simulink model "model_T_PSH_IEEE39"  (R2020b)
settings: Solver=ode3  StartTime=0.0  StopTime=300  FixedStep=Ts  RelTol=1e-3
PostLoadFcn:
  | IEEE39BusLineLength;
  | vNomHV = 345E3;fNom=60;load('Dynamicload.mat');
InitFcn:
  | IEEE39BusLineLength;
  | vNomHV = 345E3;fNom=60;load('Dynamicload.mat');
values from neighbouring files (symbols this model uses):
  At = 1.48    [MAIN_T_PSH_IEEE39.m]
  Dturb = 0.3    [MAIN_T_PSH_IEEE39.m]
  fix_mode = 1    [MAIN_T_PSH_IEEE39.m]
  Gmax = 1    [MAIN_T_PSH_IEEE39.m]
  Gmin = 0    [MAIN_T_PSH_IEEE39.m]
  Hdam = 1    [MAIN_T_PSH_IEEE39.m]
  Kd = 1    [MAIN_T_PSH_IEEE39.m]    (also in plots_T_PSH_IEEE39.m)
  max_delay_gen2pump = 20    [MAIN_T_PSH_IEEE39.m]
  max_delay_pump2hsc = 30    [MAIN_T_PSH_IEEE39.m]
  pgen_pump = Kd*Pref    (= 0.9)    [MAIN_T_PSH_IEEE39.m]
  pgen_turb = (1-Kd)*Pref    (= 0)    [MAIN_T_PSH_IEEE39.m]
  pgen_turb_gen2pump = (1-kd_gen2pump)*Pref    (= 0)    [MAIN_T_PSH_IEEE39.m]
  pgen_turb_hsc2gen = (1-kd_hsc2gen)*Pref    (= 0.36)    [MAIN_T_PSH_IEEE39.m]
  pgen_turb_pump2hsc = (1-kd_pump2hsc)*Pref    (= 0.36)    [MAIN_T_PSH_IEEE39.m]
  Pref = 0.9    [MAIN_T_PSH_IEEE39.m]    (also in MAIN_VS_PSH.m = 1)
  qNL = 0.1    [MAIN_T_PSH_IEEE39.m]
  R = 0.04    [MAIN_T_PSH_IEEE39.m]
  r = 0.31    [MAIN_T_PSH_IEEE39.m]
  Rp = 0.05    [IEEE39BusLineLength.m]
  Sn = 320E6    (= 320000000)    [MAIN_T_PSH_IEEE39.m]
  t_gen2pump = 10    [MAIN_T_PSH_IEEE39.m]
  t_hsc2gen = 150    [MAIN_T_PSH_IEEE39.m]
  t_pump2hsc = 35    [MAIN_T_PSH_IEEE39.m]
  t_sw_off = 220    [MAIN_FS_PSH_IEEE39.m]    (also in MAIN_T_PSH_IEEE39.m; MAIN_VS_PSH.m = 45)
  t_sw_on = 130    [MAIN_FS_PSH_IEEE39.m]    (also in MAIN_T_PSH_IEEE39.m; MAIN_VS_PSH.m = 35)
  Tf = 0.05    [MAIN_T_PSH_IEEE39.m]
  Tg = 0.5    [MAIN_T_PSH_IEEE39.m]
  TL_10_11_len = 14    [IEEE39BusLineLength.m]
  TL_10_13_len = 14    [IEEE39BusLineLength.m]
  TL_13_14_len = 32    [IEEE39BusLineLength.m]
  TL_14_15_len = 70    [IEEE39BusLineLength.m]
  TL_15_16_len = 31.5    [IEEE39BusLineLength.m]
  TL_16_17_len = 26    [IEEE39BusLineLength.m]
  TL_16_19_len = 61    [IEEE39BusLineLength.m]
  TL_16_21_len = 46    [IEEE39BusLineLength.m]
  TL_16_24_len = 15    [IEEE39BusLineLength.m]
  TL_17_18_len = 26    [IEEE39BusLineLength.m]
  TL_17_27_len = 59    [IEEE39BusLineLength.m]
  TL_1_2_len = 134    [IEEE39BusLineLength.m]
  TL_1_39_len = 105    [IEEE39BusLineLength.m]
  TL_21_22_len = 47    [IEEE39BusLineLength.m]
  TL_22_23_len = 33    [IEEE39BusLineLength.m]
  TL_24_23_len = 88    [IEEE39BusLineLength.m]
  TL_25_26_len = 101    [IEEE39BusLineLength.m]
  TL_26_27_len = 46.5    [IEEE39BusLineLength.m]
  TL_26_28_len = 151    [IEEE39BusLineLength.m]
  TL_26_29_len = 200    [IEEE39BusLineLength.m]
  TL_28_29_len = 48    [IEEE39BusLineLength.m]
  TL_2_25_len = 28    [IEEE39BusLineLength.m]
  TL_2_2_len = 49    [IEEE39BusLineLength.m]
  TL_3_18_len = 42    [IEEE39BusLineLength.m]
  TL_3_4_len = 53    [IEEE39BusLineLength.m]
  TL_4_14_len = 33    [IEEE39BusLineLength.m]
  TL_4_5_len = 32.5    [IEEE39BusLineLength.m]
  TL_5_6_len = 14    [IEEE39BusLineLength.m]
  TL_5_8_len = 32    [IEEE39BusLineLength.m]
  TL_6_11_len = 26.5    [IEEE39BusLineLength.m]
  TL_6_7_len = 25.5    [IEEE39BusLineLength.m]
  TL_7_8_len = 15    [IEEE39BusLineLength.m]
  TL_8_9_len = 93    [IEEE39BusLineLength.m]
  TL_9_39_len = 136    [IEEE39BusLineLength.m]
  Tr = 6.88    [MAIN_T_PSH_IEEE39.m]
  Ts = 25e-6    (= 2.5e-05)    [MAIN_FS_PSH_IEEE39.m]    (also in MAIN_T_PSH_IEEE39.m; MAIN_VS_PSH.m = 1e-07)
  Velm = 0.05    [MAIN_T_PSH_IEEE39.m]
  Vn = 18000    [MAIN_T_PSH_IEEE39.m]
undefined symbols (not defined in the file or in its folder): D1, Delta, load15, load16, load18, load20, load21, load23, load24, load25, load26, load27, load28, load29, load3, load39, load4, load7, load8
libraries: powerlib x216, sps_avr x10, simulink_extras x7, powerlib_meascontrol x5, simulink x1
(part 5 of 9)

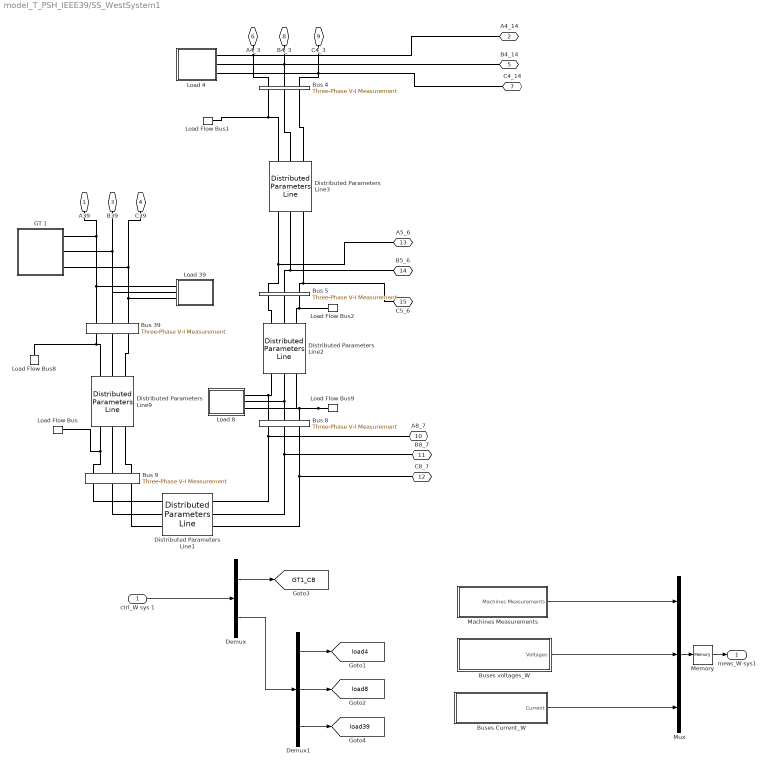
== system model_T_PSH_IEEE39/SS_WestSystem1 ==
  ctrl_W sys 1 : Inport
  Bus 39 : powerlib/Measurements/Three-Phase V-I Measurement  VoltageMeasurement=phase-to-ground  SetLabelV=on  LabelV=V_bus_39  Vpu=off  VpuLL=off  CurrentMeasurement=yes  SetLabelI=on  LabelI=I_bus_39  Ipu=off  Pbase=100e6  Vbase=345e3  OutputType=Complex  PhasorSimulation=off  PSBequivalent=0
  Bus 4 : powerlib/Measurements/Three-Phase V-I Measurement  VoltageMeasurement=phase-to-ground  SetLabelV=on  LabelV=V_bus_4  Vpu=off  VpuLL=off  CurrentMeasurement=yes  SetLabelI=on  LabelI=I_bus_4  Ipu=off  Pbase=100e6  Vbase=230e3  OutputType=Complex  PhasorSimulation=off  PSBequivalent=0
  Bus 5 : powerlib/Measurements/Three-Phase V-I Measurement  VoltageMeasurement=phase-to-ground  SetLabelV=on  LabelV=V_bus_5  Vpu=off  VpuLL=off  CurrentMeasurement=yes  SetLabelI=on  LabelI=I_bus_5  Ipu=off  Pbase=100e6  Vbase=230e3  OutputType=Complex  PhasorSimulation=off  PSBequivalent=0
  Bus 8 : powerlib/Measurements/Three-Phase V-I Measurement  VoltageMeasurement=phase-to-ground  SetLabelV=on  LabelV=V_bus_8  Vpu=off  VpuLL=off  CurrentMeasurement=yes  SetLabelI=on  LabelI=I_bus_8  Ipu=off  Pbase=100e6  Vbase=230e3  OutputType=Complex  PhasorSimulation=off  PSBequivalent=0
  Bus 9 : powerlib/Measurements/Three-Phase V-I Measurement  VoltageMeasurement=phase-to-ground  SetLabelV=on  LabelV=V_bus_9  Vpu=off  VpuLL=off  CurrentMeasurement=yes  SetLabelI=on  LabelI=I_bus_9  Ipu=off  Pbase=100e6  Vbase=230e3  OutputType=Complex  PhasorSimulation=off  PSBequivalent=0
  Buses Current_W : Subsystem
  Buses voltages_W : Subsystem
  Demux : Demux  Outputs=[1 6]
  Demux1 : Demux  Outputs=[2 2 2]
  Distributed Parameters Line1 : powerlib/Elements/Distributed Parameters Line  Phases=3  Length=TL_8_9_len  Frequency=fNom  Resistance=[2.738 10.95]/TL_8_9_len  Inductance=[0.115 0.344]/TL_8_9_len  Capacitance=[0.848e-6 0.385e-6]/TL_8_9_len  x1=[-0.000375 7.83180070356268e-09 238945.685626359 24258.781932988;-0.00035 7.68853749159509e-09 239163.697394933 22005.7375529596;-0.000325 7.5445913392716e-09 239360.465261036 19750.7384960824;-0.0003 7.39997503272177e-09 239535.971746608 17493.9850644112;-0.000275 7.25470141760213e-09 239690.201262149 15235.6777158346;-0.00025 7.10878339795517e-09 239823.140108101 12976.017046269;-0.000225 6.96223393506311e-09 239934.776476067 10715.2037718408;-0.0002 6.8150660462966e-09 240025.100449859 8453.43871105719;-0.000175 6.66729280395846e-09 240094.10400638 6190.92276696862;-0.00015 6.51892733412251e-09 240141.781016335 3927.85690932335;-0.000125 6.36998281546766e-09 240168.127244777 1664.44215671614;-0.0001 6.22047247810726e-09 240173.14035148 -599.120441267409;-7.5e-05 6.07040960241395e-09 240156.819891152 -2862.62982190919;-5e-05 5.91980751784004e-09 240119.16731347 -5125.88492721818;-2.5e-05 5.76867960173348e-09 240060.185962955 -7388.68472178954]  x2=[-0.000375 6.41970903757356e-09 248393.348574129 9449.4998144962;-0.00035 6.32122932359373e-09 248471.368448558 7108.07301672364;-0.000325 6.2221881214754e-09 248527.317659354 4766.01483880616;-0.0003 6.1225942286308e-09 248561.191236786 2423.53331589312;-0.000275 6.02245649156536e-09 248572.986172007 80.8365207378492;-0.00025 5.92178380509189e-09 248562.701417321 -2261.8674547846;-0.000225 5.82058511154051e-09 248530.337886282 -4604.37051816137;-0.0002 5.71886939996431e-09 248475.898453604 -6946.46459472579;-0.000175 5.61664570534093e-09 248399.387954912 -9287.94164613975;-0.00015 5.51392310776999e-09 248300.813186313 -11628.5936888729;-0.000125 5.41071073166657e-09 248180.182903786 -13968.2128126769;-0.0001 5.30701774495068e-09 248037.50782241 -16306.5911990532;-7.5e-05 5.20285335823298e-09 247872.800615413 -18643.521139713;-5e-05 5.09822682399658e-09 247686.075913039 -20978.7950550263;-2.5e-05 4.99314743577521e-09 247477.350301256 -23312.2055124614]  x3=[-0.000375 -2.80416857734533e-11 994.785547993016 298.958599838395;-0.00035 -2.82588220159761e-11 997.558943228101 289.569860125711;-0.000325 -2.84734481465322e-11 1000.24372950986 280.15539914373;-0.0003 -2.86855451007874e-11 1002.83966836006 270.71605313931;-0.000275 -2.88950940390642e-11 1005.34652919239 261.252660569742;-0.00025 -2.9102076348014e-11 1007.76408933299 251.766062028274;-0.000225 -2.93064736422715e-11 1010.09213404017 242.25710016944;-0.0002 -2.95082677660871e-11 1012.33045652356 232.726619634214;-0.000175 -2.970744079494e-11 1014.47885796241 223.175466974983;-0.00015 -2.990397503713e-11 1016.53714752327 213.604490580353;-0.000125 -3.00978530353495e-11 1018.50514237696 204.014540599786;-0.0001 -3.02890575682336e-11 1020.38266771482 194.406468868091;-7.5e-05 -3.047757165189e-11 1022.16955676417 184.781128829754;-5e-05 -3.0663378541408e-11 1023.8656508032 175.13937546313;-2.5e-05 -3.08464617323452e-11 1025.47079917504 165.482065204505]  x4=[-0.000375 4.48982480771432e-11 315.841922857234 -130.234658424009;-0.00035 4.48725488427444e-11 314.600450218203 -133.205545988237;-0.000325 4.48428637690998e-11 313.331032948132 -136.164601465662;-0.0003 4.48091954930093e-11 312.033783804004 -139.111562015868;-0.000275 4.47715470050838e-11 310.708818014987 -142.046165872778;-0.00025 4.47299216494798e-11 309.356253272204 -144.96815236791;-0.000225 4.46843231236019e-11 307.976209718277 -147.877261953529;-0.0002 4.4634755477775e-11 306.568809936654 -150.7732362257;-0.000175 4.45812231148839e-11 305.13417894072 -153.655817947243;-0.00015 4.45237307899826e-11 303.672444162696 -156.524751070583;-0.000125 4.44622836098719e-11 302.183735442318 -159.379780760491;-0.0001 4.43968870326456e-11 300.6681850153 -162.220653416721;-7.5e-05 4.43275468672058e-11 299.125927501596 -165.04711669654;-5e-05 4.42542692727468e-11 297.557099893435 -167.858919537134;-2.5e-05 4.41770607582085e-11 295.961841543156 -170.655812177918]  x5=0.000363923068793392  V1=ones(3,3)  V2=ones(3,3)  I1=ones(3,3)  I2=ones(3,3)  nHarmo=1  Measurements=None  Decoupling=off  VsMag0=0  VrMag0=0  VsAngle0=0  VrAngle0=0  IsMag0=0  IrMag0=0  IsAngle0=0  IrAngle0=0
  Distributed Parameters Line2 : powerlib/Elements/Distributed Parameters Line  Phases=3  Length=TL_5_8_len  Frequency=fNom  Resistance=[0.952 3.809]/TL_5_8_len  Inductance=[0.035 0.106]/TL_5_8_len  Capacitance=[0.329e-6 0.15e-6]/TL_5_8_len  x1=[-0.00015 6.51892733412251e-09 0 0;-0.000125 6.36998281546766e-09 118642.614431542 -208823.920451668;-0.0001 6.22047247810726e-09 120605.423697804 -207696.480630433;-7.5e-05 6.07040960241395e-09 122557.52009298 -206550.592006867;-5e-05 5.91980751784004e-09 124498.730220582 -205386.356365422;-2.5e-05 5.76867960173348e-09 126428.881651101 -204203.877120241]  x2=[-0.00015 6.93971136599651e-09 0 0;-0.000125 6.78863743170585e-09 127269.929121309 -203855.09967514;-0.0001 6.63696049138591e-09 129185.526033388 -202646.571246844;-7.5e-05 6.48469401785956e-09 131089.647940081 -201420.042578368;-5e-05 6.33185153631539e-09 132982.125706271 -200175.622617078;-2.5e-05 6.17844662310637e-09 134862.791231139 -198913.421899552]  x3=[-0.00015 1.24925992865406e-11 0 0;-0.000125 1.24360709657444e-11 771.064654820684 -1268.89273840881;-0.0001 1.23784380012184e-11 782.98923328193 -1261.56936239942;-7.5e-05 1.23197055122557e-11 794.844262112154 -1254.13392650475;-5e-05 1.22598787158157e-11 806.628688279148 -1246.5870911832;-2.5e-05 1.21989629260604e-11 818.341465022041 -1238.92952678831]  x4=[-0.00015 1.33899500783991e-12 0 0;-0.000125 1.07256616847881e-12 -44.3180796703685 -8.8205638210786;-0.0001 8.06042057588946e-13 -44.2330187586768 -9.23786088668168;-7.5e-05 5.39446349382905e-13 -44.1440288144991 -9.65433739206657;-5e-05 2.7280272443298e-13 -44.0511177424369 -10.0699563433819;-2.5e-05 6.13486756769849e-15 -43.9542937953889 -10.4846808229494]  x5=0.000126095202129185  V1=ones(3,3)  V2=ones(3,3)  I1=ones(3,3)  I2=ones(3,3)  nHarmo=1  Measurements=None  Decoupling=off  VsMag0=0  VrMag0=0  VsAngle0=0  VrAngle0=0  IsMag0=0  IrMag0=0  IsAngle0=0  IrAngle0=0
  Distributed Parameters Line3 : powerlib/Elements/Distributed Parameters Line  Phases=3  Length=TL_4_5_len  Frequency=fNom  Resistance=[0.952 3.809]/TL_4_5_len  Inductance=[0.04 0.121]/TL_4_5_len  Capacitance=[0.299e-6 0.136e-6]/TL_4_5_len  x1=[-0.00015 1.25269920383338e-09 0 0;-0.000125 1.10475045682001e-09 240898.71921355 -2229.53954135192;-0.0001 9.56703579483276e-10 240867.001075201 -4499.8148800452;-7.5e-05 8.08571722202861e-10 240813.887737099 -6769.69051916246;-5e-05 6.60368042906836e-10 240739.383917078 -9038.96483522477;-2.5e-05 5.12105705902926e-10 240643.496232999 -11307.4362581662]  x2=[-0.00015 6.93649042877756e-09 0 0;-0.000125 6.78534623604884e-09 240178.659570335 -8291.44191932873;-0.0001 6.63359932963387e-09 240089.841706274 -10554.6617227481;-7.5e-05 6.48126318857032e-09 239979.69767425 -12816.9440000851;-5e-05 6.32835134423504e-09 239848.237257892 -15078.0878023472;-2.5e-05 6.1748773791422e-09 239695.472134274 -17337.8922816676]  x3=[-0.00015 1.70254750551171e-11 0 0;-0.000125 1.80202007845347e-11 1054.46345997643 -65.2780377128748;-0.0001 1.9013325855524e-11 1053.80138750757 -75.2130196605794;-7.5e-05 2.00047620529739e-11 1053.04571030628 -85.1413207529886;-5e-05 2.09944213117887e-11 1052.19649549619 -95.0620591009928;-2.5e-05 2.19822157247107e-11 1051.25381850947 -104.974353487249]  x4=[-0.00015 -8.67939542222851e-12 0 0;-0.000125 -9.98973494501568e-12 258.850755039016 63.6513742271612;-0.0001 -1.12991871217834e-11 259.439132832302 61.2089665193673;-7.5e-05 -1.26076356394179e-11 260.004465741707 58.7611218772509;-5e-05 -1.39149642739563e-11 260.546703551093 56.3080577325265;-2.5e-05 -1.52210569009101e-11 261.065798095762 53.8499919805356]  x5=0.000128280941686597  V1=ones(3,3)  V2=ones(3,3)  I1=ones(3,3)  I2=ones(3,3)  nHarmo=1  Measurements=None  Decoupling=off  VsMag0=0  VrMag0=0  VsAngle0=0  VrAngle0=0  IsMag0=0  IrMag0=0  IsAngle0=0  IrAngle0=0
  Distributed Parameters Line9 : powerlib/Elements/Distributed Parameters Line  Phases=3  Length=TL_9_39_len  Frequency=fNom  Resistance=[1.19 4.761]/TL_9_39_len  Inductance=[0.079 0.237]/TL_9_39_len  Capacitance=[2.674e-6 1.216e-6]/TL_9_39_len  x1=[-0.00055 7.09289923412947e-09 101267.80708487 -227009.687509137;-0.000525 6.99866259899122e-09 103402.781539446 -226045.193356778;-0.0005 6.90380430217396e-09 105528.57116108 -225060.620563329;-0.000475 6.80833276954009e-09 107644.987124847 -224056.056584238;-0.00045 6.71225648142317e-09 109751.841438443 -223031.590650687;-0.000425 6.61558397187463e-09 111848.946958887 -221987.313761663;-0.0004 6.51832382790573e-09 113936.11740914 -220923.318675878;-0.000375 6.42048468872484e-09 116013.167394655 -219839.699903527;-0.00035 6.32207524497001e-09 118079.912419841 -218736.553697896;-0.000325 6.22310423793704e-09 120136.168904457 -217613.978046809;-0.0003 6.12358045880305e-09 122181.754199912 -216472.072663925;-0.000275 6.02351274784555e-09 124216.486605491 -215310.938979885;-0.00025 5.92290999365723e-09 126240.185384497 -214130.680133294;-0.000225 5.82178113235642e-09 128252.670780305 -212931.400961569;-0.0002 5.7201351467933e-09 130253.764032324 -211713.20799162;-0.000175 5.61798106575206e-09 132243.287391881 -210476.209430391;-0.00015 5.51532796314882e-09 134221.064138008 -209220.515155245;-0.000125 5.41218495722571e-09 136186.918593138 -207946.236704209;-0.0001 5.30856120974091e-09 138140.676138713 -206653.487266062;-7.5e-05 5.20446592515482e-09 140082.16323069 -205342.381670286;-5e-05 5.09990834981252e-09 142011.207414959 -204013.036376859;-2.5e-05 4.99489777112241e-09 143927.637342663 -202665.569465918]  x2=[-0.00055 6.87985981860704e-09 111424.440555576 -223499.219798688;-0.000525 6.86712699791032e-09 113525.87882937 -222439.159087817;-0.0005 6.85378419928722e-09 115617.233078189 -221359.34004467;-0.000475 6.83983260792228e-09 117698.317535855 -220259.858585019;-0.00045 6.8252734630765e-09 119768.947348415 -219140.812371163;-0.000425 6.81010805797731e-09 121828.938590554 -218002.300803259;-0.0004 6.79433773970369e-09 123878.108281941 -216844.425010485;-0.000375 6.77796390906648e-09 125916.274403475 -215667.287842067;-0.00035 6.76098802048401e-09 127943.255913456 -214470.993858132;-0.000325 6.74341158185284e-09 129958.872763666 -213255.64932043;-0.0003 6.72523615441389e-09 131962.945915361 -212021.362182889;-0.000275 6.70646335261371e-09 133955.297355178 -210768.242082031;-0.00025 6.68709484396111e-09 135935.75011094 -209496.400327228;-0.000225 6.66713234887902e-09 137904.128267383 -208205.949890819;-0.0002 6.64657764055167e-09 139860.256981778 -206897.005398072;-0.000175 6.6254325447671e-09 141803.962499462 -205569.683117007;-0.00015 6.603698939755e-09 143735.072169272 -204224.100948063;-0.000125 6.58137875601981e-09 145653.414458882 -202860.378413628;-0.0001 6.55847397616933e-09 147558.818970036 -201478.636647424;-7.5e-05 6.53498663473852e-09 149451.116453689 -200078.998383743;-5e-05 6.51091881800887e-09 151330.138825038 -198661.587946549;-2.5e-05 6.48627266382302e-09 153195.719178451 -197226.531238432]  x3=[-0.00055 -7.894266515009e-11 603.205379102775 -1701.19716306051;-0.000525 -7.91038421888887e-11 619.21169102253 -1695.43663133683;-0.0005 -7.92579927670378e-11 635.163000979544 -1689.52550112837;-0.000475 -7.94051031919916e-11 651.057892086235 -1683.46429749589;-0.00045 -7.95451603965517e-11 666.894952466469 -1677.25355883055;-0.000425 -7.96781519400273e-11 682.672775380972 -1670.89383680607;-0.0004 -7.98040660093404e-11 698.389959352282 -1664.38569632973;-0.000375 -7.99228914200755e-11 714.045108289242 -1657.72971549219;-0.00035 -8.00346176174725e-11 729.636831611003 -1650.92648551616;-0.000325 -8.01392346773645e-11 745.163744370547 -1643.97661070387;-0.0003 -8.02367333070594e-11 760.624467377704 -1636.88070838337;-0.000275 -8.0327104846165e-11 776.017627321662 -1629.63940885375;-0.00025 -8.04103412673589e-11 791.34185689295 -1622.2533553291;-0.000225 -8.04864351771007e-11 806.59579490489 -1614.72320388139;-0.0002 -8.05553798162895e-11 821.778086414509 -1607.04962338223;-0.000175 -8.06171690608637e-11 836.887382842889 -1599.23329544339;-0.00015 -8.06717974223453e-11 851.922342094958 -1591.27491435632;-0.000125 -8.07192600483274e-11 866.881628678702 -1583.17518703045;-0.0001 -8.07595527229052e-11 881.76391382379 -1574.93483293039;-7.5e-05 -8.07926718670503e-11 896.567875599604 -1566.55458401204;-5e-05 -8.08186145389288e-11 911.292199032663 -1558.03518465755;-2.5e-05 -8.08373784341627e-11 925.93557622342 -1549.37739160926]  x4=[-0.00055 1.12224479082197e-10 400.941440055207 -1013.32186488095;-0.000525 1.12169196582543e-10 410.473749845076 -1009.49813482846;-0.0005 1.12103950566275e-10 419.969598983085 -1005.58473531461;-0.000475 1.12028746828921e-10 429.428143993005 -1001.58201395017;-0.00045 1.11943592050513e-10 438.848544712179 -997.490326280015;-0.000425 1.11848493794989e-10 448.229964366145 -993.310035751486;-0.0004 1.11743460509528e-10 457.571569642966 -989.041513682164;-0.000375 1.11628501523792e-10 466.872530767246 -984.685139226859;-0.00035 1.11503627049103e-10 476.13202157384 -980.24129934394;-0.000325 1.11368848177535e-10 485.349219581234 -975.710388760959;-0.0003 1.11224176880926e-10 494.523306064607 -971.092809939593;-0.000275 1.11069626009817e-10 503.653466128552 -966.388973039892;-0.00025 1.1090520929231e-10 512.738888779461 -961.599295883848;-0.000225 1.10730941332849e-10 521.778766997561 -956.72420391828;-0.0002 1.10546837610921e-10 530.772297808598 -951.764130177044;-0.000175 1.10352914479683e-10 539.718682355166 -946.71951524257;-0.00015 1.1014918916451e-10 548.617125967659 -941.590807206725;-0.000125 1.09935679761462e-10 557.466838234865 -936.378461631012;-0.0001 1.09712405235678e-10 566.267033074169 -931.082941506102;-7.5e-05 1.09479385419693e-10 575.016928801383 -925.704717210712;-5e-05 1.09236641011674e-10 583.715748200174 -920.244266469823;-2.5e-05 1.08984193573583e-10 592.362718591108 -914.70207431224]  x5=0.000536835170233844  V1=ones(3,3)  V2=ones(3,3)  I1=ones(3,3)  I2=ones(3,3)  nHarmo=1  Measurements=None  Decoupling=off  VsMag0=0  VrMag0=0  VsAngle0=0  VrAngle0=0  IsMag0=0  IrMag0=0  IsAngle0=0  IrAngle0=0
  "GT 1 " : Subsystem
  Load 39 : Subsystem  SystemSampleTime=20e-3
  Load 4 : Subsystem
  Load 8 : Subsystem
  Load Flow Bus : powerlib/Measurements/Load Flow Bus  LConnTagsString=a  Phases=single  Connectors=on one side  ID=Bus-9  Vbase=345e+003  Vref=1  Vangle=0  VLF=1.022  VLFb=1  VLFc=1  angleLF=20.59  angleLFb=0  angleLFc=0
      settings: AttributesFormatString=%<ID>\n%<Vbase>V\n%<VLF>pu\n%<angleLF>deg.
  Load Flow Bus1 : powerlib/Measurements/Load Flow Bus  LConnTagsString=a  Phases=single  Connectors=on one side  ID=Bus-4  Vbase=345e+003  Vref=1  Vangle=0  VLF=0.9935  VLFb=1  VLFc=1  angleLF=19.16  angleLFb=0  angleLFc=0
      settings: AttributesFormatString=%<ID>\n%<Vbase>V\n%<VLF>pu\n%<angleLF>deg.
  Load Flow Bus2 : powerlib/Measurements/Load Flow Bus  LConnTagsString=a  Phases=single  Connectors=on one side  ID=Bus-5  Vbase=345e+003  Vref=1  Vangle=0  VLF=0.9982  VLFb=1  VLFc=1  angleLF=20.09  angleLFb=0  angleLFc=0
      settings: AttributesFormatString=%<ID>\n%<Vbase>V\n%<VLF>pu\n%<angleLF>deg.
  Load Flow Bus8 : powerlib/Measurements/Load Flow Bus  LConnTagsString=a  Phases=single  Connectors=on one side  ID=Bus-39  Vbase=345000  Vref=1.03  Vangle=0  VLF=1.029  VLFb=1  VLFc=1  angleLF=21.84  angleLFb=0  angleLFc=0
      settings: AttributesFormatString=%<ID>\n%<Vbase>V\n%<VLF>pu\n%<angleLF>deg.
  Load Flow Bus9 : powerlib/Measurements/Load Flow Bus  LConnTagsString=a  Phases=single  Connectors=on one side  ID=Bus-8  Vbase=345e+003  Vref=1  Vangle=0  VLF=0.9916  VLFb=1  VLFc=1  angleLF=18.81  angleLFb=0  angleLFc=0
      settings: AttributesFormatString=%<ID>\n%<Vbase>V\n%<VLF>pu\n%<angleLF>deg.
  Machines Measurements : Subsystem
      mask Display: disp('Machines Measurements')
  Memory : Memory
  Mux : Mux  Inputs=3
  A39 : PMIOPort  Side=Right
  A4_14 : PMIOPort  Port=2  Side=Left
  B39 : PMIOPort  Port=3  Side=Right
  C39 : PMIOPort  Port=4  Side=Right
  B4_14 : PMIOPort  Port=5  Side=Left
  A4_3 : PMIOPort  Port=6  Side=Right
  C4_14 : PMIOPort  Port=7  Side=Left
  B4_3 : PMIOPort  Port=8  Side=Right
  C4_3 : PMIOPort  Port=9  Side=Right
  A8_7 : PMIOPort  Port=10  Side=Left
  B8_7 : PMIOPort  Port=11  Side=Left
  C8_7 : PMIOPort  Port=12  Side=Left
  A5_6 : PMIOPort  Port=13  Side=Right
  B5_6 : PMIOPort  Port=14  Side=Right
  C5_6 : PMIOPort  Port=15  Side=Right
  meas_W sys1 : Outport
  tag scope: GT1_CB=global, load39=global, load4=global, load8=global
  wires:
  ctrl_W sys 1/1 -> Demux/1
  Mux/1 -> Memory/1
  Memory/1 -> meas_W sys1/1
  Buses voltages_W/1(Voltages) -> Mux/2
  Machines Measurements/1(Machines Measurements) -> Mux/1
  Buses Current_W/1(Current) -> Mux/3
  Demux/1 -> [GT1_CB]
  Demux/2 -> Demux1/1
  Demux1/2 -> [load8]
  Demux1/1 -> [load4]
  Demux1/3 -> [load39]
  connections:
  Distributed Parameters Line9/LConn3 -- Bus 9/RConn3
  Distributed Parameters Line9/LConn2 -- Bus 9/RConn2
  Bus 9/RConn1 -- Distributed Parameters Line9/LConn1 -- Load Flow Bus/LConn1
  Load Flow Bus9/LConn1 -- Distributed Parameters Line2/LConn3 -- Load 8/LConn3 -- Bus 8/RConn3
  Load 8/LConn2 -- Distributed Parameters Line2/LConn2 -- Bus 8/RConn2
  Load 8/LConn1 -- Distributed Parameters Line2/LConn1 -- Bus 8/RConn1
  Bus 8/LConn3 -- Distributed Parameters Line1/LConn1 -- C8_7/RConn1
  Bus 8/LConn2 -- Distributed Parameters Line1/LConn2 -- B8_7/RConn1
  A8_7/RConn1 -- Distributed Parameters Line1/LConn3 -- Bus 8/LConn1
  Bus 5/RConn3 -- C5_6/RConn1 -- Distributed Parameters Line3/RConn1
  Bus 5/RConn2 -- B5_6/RConn1 -- Distributed Parameters Line3/RConn2
  Bus 5/RConn1 -- Distributed Parameters Line3/RConn3 -- A5_6/RConn1
  "GT 1 "/RConn3 -- Bus 39/RConn3 -- Load 39/LConn3 -- C39/RConn1
  "GT 1 "/RConn2 -- Load 39/LConn2 -- Bus 39/RConn2 -- B39/RConn1
  Bus 39/RConn1 -- "GT 1 "/RConn1 -- A39/RConn1 -- Load 39/LConn1
  Load Flow Bus8/LConn1 -- Distributed Parameters Line9/RConn1 -- Bus 39/LConn1
  Distributed Parameters Line9/RConn2 -- Bus 39/LConn2
  Distributed Parameters Line9/RConn3 -- Bus 39/LConn3
  Bus 9/LConn1 -- Distributed Parameters Line1/RConn3
  Distributed Parameters Line1/RConn2 -- Bus 9/LConn2
  Bus 9/LConn3 -- Distributed Parameters Line1/RConn1
  Distributed Parameters Line2/RConn1 -- Bus 5/LConn1
  Distributed Parameters Line2/RConn2 -- Bus 5/LConn2
  Load Flow Bus2/LConn1 -- Distributed Parameters Line2/RConn3 -- Bus 5/LConn3
  Load Flow Bus1/LConn1 -- Distributed Parameters Line3/LConn3 -- Bus 4/LConn1
  Bus 4/LConn2 -- Distributed Parameters Line3/LConn2
  Bus 4/LConn3 -- Distributed Parameters Line3/LConn1
  B4_3/RConn1 -- B4_14/RConn1 -- Load 4/LConn2 -- Bus 4/RConn2
  A4_3/RConn1 -- A4_14/RConn1 -- Load 4/LConn1 -- Bus 4/RConn1
  C4_3/RConn1 -- C4_14/RConn1 -- Load 4/LConn3 -- Bus 4/RConn3

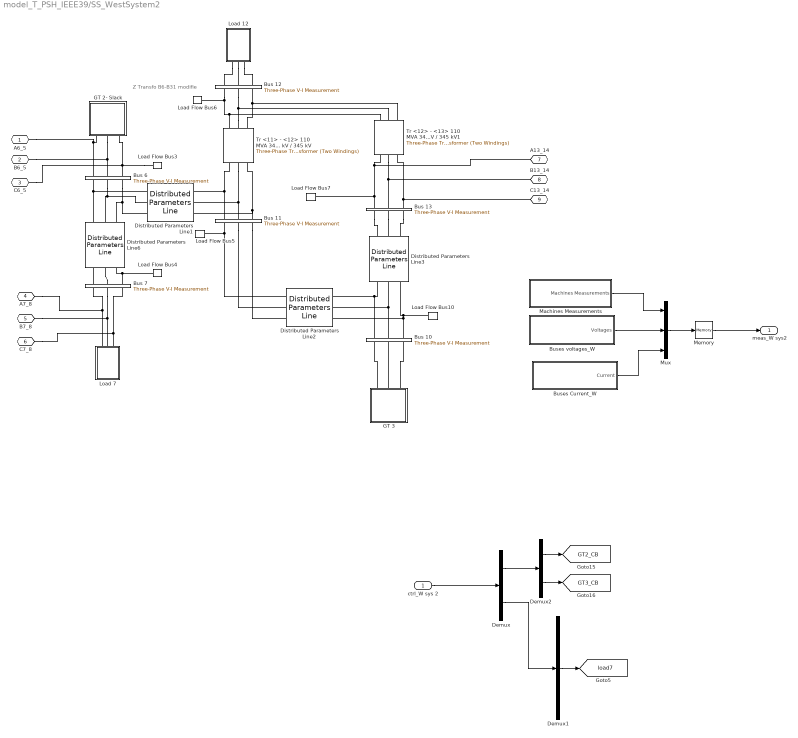
== system model_T_PSH_IEEE39/SS_WestSystem2 ==
  note: Z Transfo B6-B31 modifie
  ctrl_W sys 2 : Inport
  Bus 10 : powerlib/Measurements/Three-Phase V-I Measurement  VoltageMeasurement=phase-to-ground  SetLabelV=on  LabelV=V_bus_10  Vpu=off  VpuLL=off  CurrentMeasurement=yes  SetLabelI=on  LabelI=I_bus_10  Ipu=off  Pbase=100e6  Vbase=230e3  OutputType=Complex  PhasorSimulation=off  PSBequivalent=0
  Bus 11 : powerlib/Measurements/Three-Phase V-I Measurement  VoltageMeasurement=phase-to-ground  SetLabelV=on  LabelV=V_bus_11  Vpu=off  VpuLL=off  CurrentMeasurement=yes  SetLabelI=on  LabelI=I_bus_11  Ipu=off  Pbase=100e6  Vbase=230e3  OutputType=Complex  PhasorSimulation=off  PSBequivalent=0
  Bus 12 : powerlib/Measurements/Three-Phase V-I Measurement  VoltageMeasurement=phase-to-ground  SetLabelV=on  LabelV=V_bus_12  Vpu=off  VpuLL=off  CurrentMeasurement=yes  SetLabelI=on  LabelI=I_bus_12  Ipu=off  Pbase=100e6  Vbase=230e3  OutputType=Complex  PhasorSimulation=off  PSBequivalent=0
  Bus 13 : powerlib/Measurements/Three-Phase V-I Measurement  VoltageMeasurement=phase-to-ground  SetLabelV=on  LabelV=V_bus_13  Vpu=off  VpuLL=off  CurrentMeasurement=yes  SetLabelI=on  LabelI=I_bus_13  Ipu=off  Pbase=100e6  Vbase=230e3  OutputType=Complex  PhasorSimulation=off  PSBequivalent=0
  Bus 6 : powerlib/Measurements/Three-Phase V-I Measurement  VoltageMeasurement=phase-to-ground  SetLabelV=on  LabelV=V_bus_6  Vpu=off  VpuLL=off  CurrentMeasurement=yes  SetLabelI=on  LabelI=I_bus_6  Ipu=off  Pbase=100e6  Vbase=230e3  OutputType=Complex  PhasorSimulation=off  PSBequivalent=0
  Bus 7 : powerlib/Measurements/Three-Phase V-I Measurement  VoltageMeasurement=phase-to-ground  SetLabelV=on  LabelV=V_bus_7  Vpu=off  VpuLL=off  CurrentMeasurement=yes  SetLabelI=on  LabelI=I_bus_7  Ipu=off  Pbase=100e6  Vbase=230e3  OutputType=Complex  PhasorSimulation=off  PSBequivalent=0
  Buses Current_W : Subsystem
  Buses voltages_W : Subsystem
  Demux : Demux  Outputs=[2 2]
  Demux1 : Demux  Outputs=[2 ]
  Demux2 : Demux  Outputs=2
  Distributed Parameters Line1 : powerlib/Elements/Distributed Parameters Line  Phases=3  Length=TL_6_11_len  Frequency=fNom  Resistance=[0.833 3.333]/TL_6_11_len  Inductance="[0.026  0.078]/TL_6_11_len"  Capacitance=[0.31e-6 0.141e-6]/TL_6_11_len  x1=[-0.000125 6.75577875850772e-09 0 0;-0.0001 6.59029012801169e-09 134309.371118129 -199264.945938064;-7.5e-05 6.42421610984077e-09 136181.394846462 -197990.276944669;-5e-05 6.25757145564951e-09 138041.32215589 -196698.021310076;-2.5e-05 6.09037096777966e-09 139888.987836916 -195388.293819903]  x2=[-0.000125 -1.24002466010301e-08 0 0;-0.0001 -1.25301492699702e-08 139717.424572789 -195819.97961294;-7.5e-05 -1.26589389386017e-08 141556.741164788 -194494.495667552;-5e-05 -1.27866041670813e-08 143383.483868541 -193151.735596473;-2.5e-05 -1.29131336154454e-08 145197.490422199 -191791.818671416]  x3=[-0.000125 -1.87906057087571e-10 0 0;-0.0001 -1.94031871091992e-10 846.127228422234 -1211.89602561571;-7.5e-05 -2.0014045006371e-10 857.511398363917 -1203.86769961341;-5e-05 -2.06231251403422e-10 868.81939918498 -1195.73243912115;-2.5e-05 -2.12303734090935e-10 880.050226443407 -1187.4909667598]  x4=[-0.000125 1.81889724805271e-10 0 0;-0.0001 1.87612525041832e-10 74.9879650040595 -165.37585370086;-7.5e-05 1.93318660449125e-10 76.5430994436869 -164.661825729295;-5e-05 1.99007624175209e-10 78.0914348826419 -163.933171542278;-2.5e-05 2.04678910893431e-10 79.6328337888181 -163.189955863086]  x5=0.000104871349757691  V1=ones(3,3)  V2=ones(3,3)  I1=ones(3,3)  I2=ones(3,3)  nHarmo=1  Measurements=None  Decoupling=off  VsMag0=0  VrMag0=0  VsAngle0=0  VrAngle0=0  IsMag0=0  IrMag0=0  IsAngle0=0  IrAngle0=0
  Distributed Parameters Line2 : powerlib/Elements/Distributed Parameters Line  Phases=3  Length=TL_10_11_len  Frequency=fNom  Resistance=[0.476 1.904]/TL_10_11_len  Inductance="[0.014  0.04]/TL_10_11_len"  Capacitance=[0.162e-6 0.074e-6]/TL_10_11_len  x1=[-7.5e-05 -1.26587332431561e-08 0 0;-5e-05 -1.27864670266328e-08 143383.483868541 -193151.735596473;-2.5e-05 -1.29130650421756e-08 145197.490422199 -191791.818671416]  x2=[-7.5e-05 -2.31876988074677e-08 0 0;-5e-05 -2.33137239864337e-08 146762.32836265 -191505.564377099;-2.5e-05 -2.34376783056329e-08 148560.67060161 -190113.87669968]  x3=[-7.5e-05 -1.13343003514613e-10 0 0;-5e-05 -1.20004737613399e-10 847.627690256735 -1267.27349806871;-2.5e-05 -1.26655812197512e-10 859.533706800166 -1259.22857632917]  x4=[-7.5e-05 6.61796513204937e-11 0 0;-5e-05 7.2439173232445e-11 126.421029639265 -48.4727009085393;-2.5e-05 7.86922606781792e-11 126.872113693026 -47.2791251432981]  x5=5.44058820349418e-05  V1=ones(3,3)  V2=ones(3,3)  I1=ones(3,3)  I2=ones(3,3)  nHarmo=1  Measurements=None  Decoupling=off  VsMag0=0  VrMag0=0  VsAngle0=0  VrAngle0=0  IsMag0=0  IrMag0=0  IsAngle0=0  IrAngle0=0
  Distributed Parameters Line3 : powerlib/Elements/Distributed Parameters Line  Phases=3  Length=TL_10_13_len  Frequency=fNom  Resistance=[0.476 1.904]/TL_10_13_len  Inductance=[0.014 0.04]/TL_10_13_len  Capacitance=[0.162e-6 0.074e-6]/TL_10_13_len  x1=[-7.5e-05 -1.88339482025469e-08 0 0;-5e-05 -1.89556448338268e-08 239362.923709733 -26461.068481927;-2.5e-05 -1.90756577151292e-08 239102.901113639 -28715.7935898655]  x2=[-7.5e-05 -2.31913353322025e-08 0 0;-5e-05 -2.33173613189625e-08 239229.847897969 -31347.1224920588;-2.5e-05 -2.34413161228668e-08 238923.782134671 -33600.3763944065]  x3=[-7.5e-05 -2.62101767642871e-11 0 0;-5e-05 -2.90902879880613e-11 1729.39624743813 -190.341770768129;-2.5e-05 -3.19678152442535e-11 1727.52552375613 -206.632261965388]  x4=[-7.5e-05 -2.95767333047303e-11 0 0;-5e-05 -2.70591342112524e-11 -101.588549005481 8.53839191220045;-2.5e-05 -2.45391315690152e-11 -101.503590188679 9.49551795694111]  x5=5.44058820349418e-05  V1=ones(3,3)  V2=ones(3,3)  I1=ones(3,3)  I2=ones(3,3)  nHarmo=1  Measurements=None  Decoupling=off  VsMag0=0  VrMag0=0  VsAngle0=0  VrAngle0=0  IsMag0=0  IrMag0=0  IsAngle0=0  IrAngle0=0
  Distributed Parameters Line6 : powerlib/Elements/Distributed Parameters Line  Phases=3  Length=TL_6_7_len  Frequency=fNom  Resistance=[0.714 2.857]/TL_6_7_len  Inductance=[0.029 0.087]/TL_6_7_len  Capacitance=[0.252e-6 0.114e-6]/TL_6_7_len  x1=[-0.0001 6.59029012801169e-09 239723.190825161 -16682.8543855798;-7.5e-05 6.42421610984077e-09 239555.306959631 -18941.4089875009;-5e-05 6.25757145564951e-09 239366.144406604 -21198.2811039545;-2.5e-05 6.09037096777966e-09 239155.719968592 -23453.2702665099]  x2=[-0.0001 6.91021686434902e-09 239820.384601578 -3394.66379905177;-7.5e-05 6.76743660664417e-09 239777.732816185 -5654.72447714792;-5e-05 6.62405522608992e-09 239713.782586145 -7914.28286991982;-2.5e-05 6.48008545864954e-09 239628.539591886 -10173.138270326]  x3=[-0.0001 -6.58530595985299e-11 -502.308537788336 50.0744676105942;-7.5e-05 -6.59005728890104e-11 -501.814306051506 54.8063466055729;-5e-05 -6.59422325095631e-11 -501.275500266472 59.5333573839503;-2.5e-05 -6.59780347597398e-11 -500.692168293079 64.255080065297]  x4=[-0.0001 7.78006133269107e-11 1914.64083956189 -86.409403369201;-7.5e-05 7.74608547902419e-11 1913.74139694153 -104.450336754876;-5e-05 7.71142157325641e-11 1912.67196474484 -122.481992257698;-2.5e-05 7.67607269443628e-11 1911.43263796498 -140.502768201765]  x5=9.9589156036187e-05  V1=ones(3,3)  V2=ones(3,3)  I1=ones(3,3)  I2=ones(3,3)  nHarmo=1  Measurements=None  Decoupling=off  VsMag0=0  VrMag0=0  VsAngle0=0  VrAngle0=0  IsMag0=0  IrMag0=0  IsAngle0=0  IrAngle0=0
  GT 2- Slack : Subsystem
  GT 3 : Subsystem
  Load 12 : Subsystem
  Load 7 : Subsystem
  Load Flow Bus10 : powerlib/Measurements/Load Flow Bus  LConnTagsString=a  Phases=single  Connectors=on one side  ID=Bus-10  Vbase=345e+003  Vref=1  Vangle=0  VLF=1.011  VLFb=1  VLFc=1  angleLF=22.22  angleLFb=0  angleLFc=0
      settings: AttributesFormatString=%<ID>\n%<Vbase>V\n%<VLF>pu\n%<angleLF>deg.
  Load Flow Bus3 : powerlib/Measurements/Load Flow Bus  LConnTagsString=a  Phases=single  Connectors=on one side  ID=Bus-6  Vbase=345e+003  Vref=1  Vangle=0  VLF=1.003  VLFb=1  VLFc=1  angleLF=20.92  angleLFb=0  angleLFc=0
      settings: AttributesFormatString=%<ID>\n%<Vbase>V\n%<VLF>pu\n%<angleLF>deg.
  Load Flow Bus4 : powerlib/Measurements/Load Flow Bus  LConnTagsString=a  Phases=single  Connectors=on one side  ID=Bus-7  Vbase=345e+003  Vref=1  Vangle=0  VLF=0.9928  VLFb=1  VLFc=1  angleLF=19.19  angleLFb=0  angleLFc=0
      settings: AttributesFormatString=%<ID>\n%<Vbase>V\n%<VLF>pu\n%<angleLF>deg.
  Load Flow Bus5 : powerlib/Measurements/Load Flow Bus  LConnTagsString=a  Phases=single  Connectors=on one side  ID=Bus-11  Vbase=345e+003  Vref=1  Vangle=0  VLF=1.007  VLFb=1  VLFc=1  angleLF=21.76  angleLFb=0  angleLFc=0
      settings: AttributesFormatString=%<ID>\n%<Vbase>V\n%<VLF>pu\n%<angleLF>deg.
  Load Flow Bus6 : powerlib/Measurements/Load Flow Bus  LConnTagsString=a  Phases=single  Connectors=on one side  ID=Bus-12  Vbase=345e+003  Vref=1  Vangle=0  VLF=0.996  VLFb=1  VLFc=1  angleLF=51.6  angleLFb=0  angleLFc=0
      settings: AttributesFormatString=%<ID>\n%<Vbase>V\n%<VLF>pu\n%<angleLF>deg.
  Load Flow Bus7 : powerlib/Measurements/Load Flow Bus  LConnTagsString=a  Phases=single  Connectors=on one side  ID=Bus-13  Vbase=345e+003  Vref=1  Vangle=0  VLF=1.007  VLFb=1  VLFc=1  angleLF=21.59  angleLFb=0  angleLFc=0
      settings: AttributesFormatString=%<ID>\n%<Vbase>V\n%<VLF>pu\n%<angleLF>deg.
  Machines Measurements : Subsystem
      mask Display: disp('Machines Measurements')
  Memory : Memory
  Mux : Mux  Inputs=3
  Tr <11> - <12> 110 MVA 345 kV / 345 kV : powerlib/Elements/Three-Phase Transformer (Two Windings)  Winding1Connection=Delta (D1)  Winding2Connection=Yg  CoreType=Three single-phase transformers  SetSaturation=off  Hysteresis=off  DataFile='hysteresis'  SetInitialFlux=off  Measurements=None  UNITS=pu  NominalPower=[ 110e6 fNom]  Winding1="[345e3 0.0016*110/100/2   0.0435*110/100/2]"  Winding2="[ 1.006*345e3 0.0016*110/100/2   0.0435*110/100/2]"  Rm=500  Lm=500  L0=0.5  Saturation="[ 0,0  ;  0.005,1.2  ;  1.0,1.4 ]"  InitialFluxes=[ 0.8 , -0.8 , 0.7 ]  BreakLoop=off  DiscreteSolver=Trapezoidal iterative  DataType=off  TransfoNumber=0
  Tr <12> - <13> 110 MVA 345 kV / 345 kV1 : powerlib/Elements/Three-Phase Transformer (Two Windings)  Winding1Connection=Delta (D1)  Winding2Connection=Yg  CoreType=Three single-phase transformers  SetSaturation=off  Hysteresis=off  DataFile='hysteresis'  SetInitialFlux=off  Measurements=None  UNITS=pu  NominalPower=[ 110e6 fNom]  Winding1="[ 345e3  0.0016*110/100/2   0.0435*110/100/2]"  Winding2="[ 1.006*345e3  0.0016*110/100/2   0.0435*110/100/2]"  Rm=500  Lm=500  L0=0.5  Saturation="[ 0,0  ;  0.005,1.2  ;  1.0,1.4 ]"  InitialFluxes=[ 0.8 , -0.8 , 0.7 ]  BreakLoop=off  DiscreteSolver=Trapezoidal iterative  DataType=off  TransfoNumber=0
  A6_5 : PMIOPort  Side=Left
  B6_5 : PMIOPort  Port=2  Side=Left
  C6_5 : PMIOPort  Port=3  Side=Left
  A7_8 : PMIOPort  Port=4  Side=Left
  B7_8 : PMIOPort  Port=5  Side=Left
  C7_8 : PMIOPort  Port=6  Side=Left
  A13_14 : PMIOPort  Port=7  Side=Right
  B13_14 : PMIOPort  Port=8  Side=Right
  C13_14 : PMIOPort  Port=9  Side=Right
  meas_W sys2 : Outport
  tag scope: GT2_CB=global, GT3_CB=global, load7=global
  wires:
  Mux/1 -> Memory/1
  Memory/1 -> meas_W sys2/1
  Buses voltages_W/1(Voltages) -> Mux/2
  Machines Measurements/1(Machines Measurements) -> Mux/1
  Buses Current_W/1(Current) -> Mux/3
  ctrl_W sys 2/1 -> Demux/1
  Demux/2 -> Demux1/1
  Demux/1 -> Demux2/1
  Demux2/1 -> [GT2_CB]
  Demux2/2 -> [GT3_CB]
  Demux1/1 -> [load7]
  connections:
  Bus 7/RConn3 -- Distributed Parameters Line6/RConn1 -- Load Flow Bus4/LConn1
  Load Flow Bus3/LConn1 -- C6_5/RConn1 -- GT 2- Slack/RConn3 -- Bus 6/RConn3
  GT 2- Slack/RConn2 -- B6_5/RConn1 -- Bus 6/RConn2
  GT 2- Slack/RConn1 -- Bus 6/RConn1 -- A6_5/RConn1
  Bus 6/LConn3 -- Distributed Parameters Line1/LConn3 -- Distributed Parameters Line6/LConn1
  Bus 6/LConn2 -- Distributed Parameters Line1/LConn2 -- Distributed Parameters Line6/LConn2
  Bus 6/LConn1 -- Distributed Parameters Line1/LConn1 -- Distributed Parameters Line6/LConn3
  Bus 13/RConn3 -- Tr <12> - <13> 110 MVA 345 kV / 345 kV1/LConn3 -- C13_14/RConn1
  Tr <12> - <13> 110 MVA 345 kV / 345 kV1/LConn2 -- Bus 13/RConn2 -- B13_14/RConn1
  Load Flow Bus7/LConn1 -- Bus 13/RConn1 -- Tr <12> - <13> 110 MVA 345 kV / 345 kV1/LConn1 -- A13_14/RConn1
  Load 12/LConn3 -- Bus 12/RConn3
  Load 12/LConn2 -- Bus 12/RConn2
  Load 12/LConn1 -- Bus 12/RConn1
  Bus 12/LConn3 -- Tr <11> - <12> 110 MVA 345 kV / 345 kV/RConn3 -- Tr <12> - <13> 110 MVA 345 kV / 345 kV1/RConn3
  Tr <11> - <12> 110 MVA 345 kV / 345 kV/RConn2 -- Bus 12/LConn2 -- Tr <12> - <13> 110 MVA 345 kV / 345 kV1/RConn2
  Load Flow Bus6/LConn1 -- Tr <12> - <13> 110 MVA 345 kV / 345 kV1/RConn1 -- Tr <11> - <12> 110 MVA 345 kV / 345 kV/RConn1 -- Bus 12/LConn1
  Bus 11/RConn3 -- Tr <11> - <12> 110 MVA 345 kV / 345 kV/LConn3 -- Distributed Parameters Line1/RConn3
  Tr <11> - <12> 110 MVA 345 kV / 345 kV/LConn2 -- Distributed Parameters Line1/RConn2 -- Bus 11/RConn2
  Tr <11> - <12> 110 MVA 345 kV / 345 kV/LConn1 -- Bus 11/RConn1 -- Distributed Parameters Line1/RConn1
  Bus 11/LConn3 -- Distributed Parameters Line2/LConn3
  Bus 11/LConn2 -- Distributed Parameters Line2/LConn2
  Load Flow Bus5/LConn1 -- Distributed Parameters Line2/LConn1 -- Bus 11/LConn1
  Bus 10/RConn3 -- Distributed Parameters Line2/RConn3 -- Distributed Parameters Line3/RConn1 -- Load Flow Bus10/LConn1
  Distributed Parameters Line2/RConn2 -- Distributed Parameters Line3/RConn2 -- Bus 10/RConn2
  Bus 10/RConn1 -- Distributed Parameters Line3/RConn3 -- Distributed Parameters Line2/RConn1
  GT 3/RConn3 -- Bus 10/LConn3
  GT 3/RConn2 -- Bus 10/LConn2
  GT 3/RConn1 -- Bus 10/LConn1
  Bus 7/LConn1 -- A7_8/RConn1 -- Load 7/LConn1
  Bus 7/LConn2 -- Load 7/LConn2 -- B7_8/RConn1
  Bus 7/LConn3 -- C7_8/RConn1 -- Load 7/LConn3
  Distributed Parameters Line6/RConn2 -- Bus 7/RConn2
  Bus 7/RConn1 -- Distributed Parameters Line6/RConn3
  Bus 13/LConn1 -- Distributed Parameters Line3/LConn3
  Bus 13/LConn2 -- Distributed Parameters Line3/LConn2
  Bus 13/LConn3 -- Distributed Parameters Line3/LConn1
